simulink model "ModelHeatTreatment"  (R2020b)
settings: Solver=FixedStepAuto  StartTime=0.0  StopTime=Inf  FixedStep=0.010  RelTol=1e-3
settings Model: Creator=kaebi  LastModifiedBy=kaebi
settings OptimizationCC: DefaultParameterBehavior=Inlined  LocalBlockOutputs=off
settings RTWCC: Description=TwinCAT GRT Target  SystemTargetFile=TwinCatGrt.tlc  GenCodeOnly=on  TemplateMakefile=tcgrt_msbuild.tmf  TargetLang=C++
settings STFCustomTargetCC: TargetLangStandard=C++03 (ISO)  ConcurrentExecutionCompliant=off  CombineOutputUpdateFcns=on  CodeInterfacePackaging=Reusable function  GRTInterface=off  GenerateAllocFcn=on  SystemTargetFile=TwinCatGrt.tlc
settings GRTTargetCC: TargetLangStandard=C++03 (ISO)  ParMdlRefBuildCompliant=off  CompOptLevelCompliant=off  ConcurrentExecutionCompliant=off  MatFileLogging=off  CodeInterfacePackaging=Reusable function  GenerateAllocFcn=on  UseToolchainInfoCompliant=off  ExtModeMexFile=TcExtModeClient

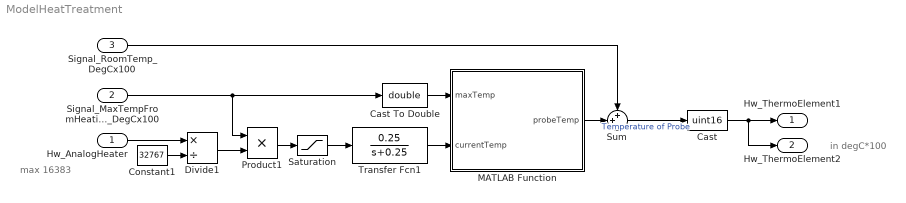
== system ModelHeatTreatment ==
  note: max 16383
  note: in degC*100
  Hw_AnalogHeater : Inport  OutDataTypeStr=uint16
  Signal_MaxTempFromHeating_DegCx100 : Inport  Port=2  OutDataTypeStr=uint16
  Signal_RoomTemp_DegCx100 : Inport  Port=3  OutDataTypeStr=uint16
  Cast : DataTypeConversion  OutDataTypeStr=uint16
  Cast To Double : DataTypeConversion  OutDataTypeStr=double
  Constant1 : Constant  Value=32767
  Divide1 : Product  Inputs=*/  OutDataTypeStr=double
  MATLAB Function : MATLAB Function  TreatAsAtomicUnit=on
  Product1 : Product
  Saturation : Saturate  UpperLimit=inf  LowerLimit=0
  Sum : Sum  Inputs=++|
  Transfer Fcn1 : TransferFcn  Numerator=[0.25]  Denominator=[1 0.25]
  Hw_ThermoElement1 : Outport
  Hw_ThermoElement2 : Outport  Port=2
  wires:
  Signal_RoomTemp_DegCx100/1 -> Sum/1
  Sum/1 -> Cast/1  "Temperature of Probe"
  MATLAB Function/1(probeTemp) -> Sum/2
  Constant1/1 -> Divide1/2
  Divide1/1 -> Product1/2
  Product1/1 -> Saturation/1
  Transfer Fcn1/1 -> MATLAB Function/2(currentTemp)
  Hw_AnalogHeater/1 -> Divide1/1
  Cast/1 -> Hw_ThermoElement2/1, Hw_ThermoElement1/1
  Saturation/1 -> Transfer Fcn1/1
  Signal_MaxTempFromHeating_DegCx100/1 -> Product1/1, Cast To Double/1
  Cast To Double/1 -> MATLAB Function/1(maxTemp)

== matlab function ModelHeatTreatment/MATLAB Function ==
  data: maxTemp input; probeTemp output; currentTemp input
function probeTemp = TemperatureModel(maxTemp, currentTemp)

if (currentTemp < 0)
    currentTemp = 0;
elseif (currentTemp > maxTemp)
    currentTemp = maxTemp;
end


probeTemp = currentTemp;
